simulink model "sim_dcmotor_model"  (R2020b)
settings: Solver=ode1  StartTime=0.0  StopTime=30  FixedStep=0.01  RelTol=1e-3
settings Model: Creator=ONLY-GOD  LastModifiedBy=ONLY-GOD
settings OptimizationCC: EnhancedBackFolding=on  PassReuseOutputArgsAs=Individual arguments  ZeroExternalMemoryAtStartup=off  ZeroInternalMemoryAtStartup=off  MaxStackSize=64  OptimizeBlockOrder=speed  DifferentSizesBufferReuse=on  OptimizationCustomize=off  EfficientTunableParamExpr=on
settings DebuggingCC: ParameterTunabilityLossMsg=error
settings HardwareCC: ProdBitPerPointer=32  ProdBitPerSizeT=32  ProdBitPerPtrDiffT=32  ProdLargestAtomicFloat=None  ProdIntDivRoundTo=Undefined  ProdEndianess=Unspecified  ProdWordSize=32  ProdHWDeviceType=Generic->Unspecified (assume 32-bit Generic)
settings SFSimCC: MATLABDynamicMemAlloc=off
settings RTWCC: Description=Embedded Coder  SystemTargetFile=ert.tlc  HardwareBoard=Robot Operating System (ROS)  TLCOptions="-aInlineSetEventsForThisBaseRateFcn=TLC_FALSE -aSuppressMultiTaskScheduler=TLC_FALSE  -aRateBasedStepFcn=0"  TemplateMakefile=ert_default_tmf  Toolchain=Catkin  TargetLang=C++
settings CodeAppCC: ForceParamTrailComments=on  IgnoreCustomStorageClasses=off  OperatorAnnotations=on  SimulinkDataObjDesc=on  SFDataObjDesc=on  InsertBlockDesc=on

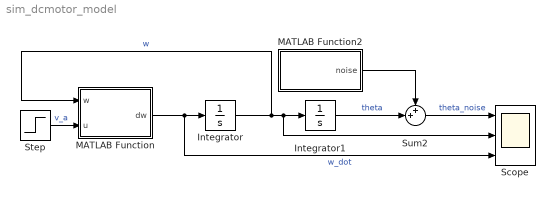
== system sim_dcmotor_model ==
  Integrator : Integrator
  Integrator1 : Integrator
  MATLAB Function : MATLAB Function  TreatAsAtomicUnit=on
  MATLAB Function2 : MATLAB Function  TreatAsAtomicUnit=on
  Scope : Scope  NumInputPorts=3
  Step : Step  After=20  SampleTime=0
  Sum2 : Sum  Inputs=++|
  wires:
  MATLAB Function/1(dw) -> Scope/3, Integrator/1  "w_dot"
  MATLAB Function2/1(noise) -> Sum2/1
  Sum2/1 -> Scope/1  "theta_noise"
  Integrator/1 -> Scope/2, Integrator1/1, MATLAB Function/1(w)  "w"
  Integrator1/1 -> Sum2/2  "theta"
  Step/1 -> MATLAB Function/2(u)  "v_a"

== matlab function sim_dcmotor_model/MATLAB Function2 ==
  data: noise output
function noise = fcn

noise = 0.1*randn;

== matlab function sim_dcmotor_model/MATLAB Function ==
  settings: updateMethod=DISCRETE
  data: w input; u input; dw output
function dw = dcmotor(w,u)
% Lamped parameters found from real dc motor
a = 27.65;
b = 17.35;
c = 5.63;
dw = -a*w+b*u-c*sign(w) + 1e-4*randn;
